simulink model "model"  (R2017a)
settings: Solver=ode45  StartTime=0.0  StopTime=25  MaxStep=0.005  MinStep=0.00001  RelTol=1e-4
settings Model: Creator=wangc  LastModifiedBy=wangc

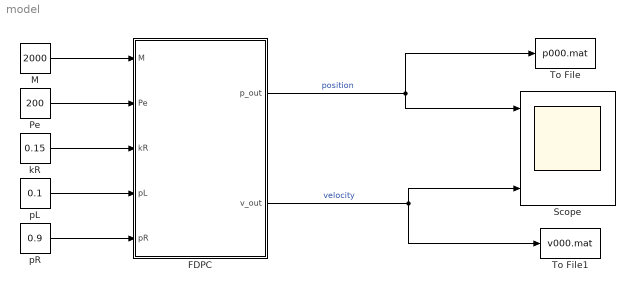
== system model ==
  FDPC : Stateflow chart  TreatAsAtomicUnit=on
  M : Constant  Value=2000
  Pe : Constant  Value=200
  Scope : Scope  NumInputPorts=3
  To File : ToFile  Filename=p000.mat  MatrixName=p  SaveFormat=Timeseries
  To File1 : ToFile  Filename=v000.mat  MatrixName=v  SaveFormat=Timeseries
  kR : Constant  Value=0.15
  pL : Constant  Value=0.1
  pR : Constant  Value=0.9
  wires:
  FDPC/2(v_out) -> To File1/1, Scope/3  "velocity"
  FDPC/1(p_out) -> To File/1, Scope/1  "position"
  M/1 -> FDPC/1(M)
  Pe/1 -> FDPC/2(Pe)
  kR/1 -> FDPC/3(kR)
  pL/1 -> FDPC/4(pL)
  pR/1 -> FDPC/5(pR)

== stateflow chart model/FDPC ==
  settings: updateMethod=CONTINUOUS  executeAtInitialization=1  initializeOutput=1
  state drivf=driv(vt, dirt, Pet) [function]
    (default) -> (junction 54) : {drivf=0.95*Pet*dirt/(vt+0.00005);}
  state system_mode_1 [group]
    state drivL
      du:
      % derivatives
      p_dot = v;
      v_dot = driv(v, dir, Pe)/M-9.81*kR;
      % outputs
      p_out = p;
      v_out = v;
    state drivL1
      du:
      % derivatives
      p_dot = v;
      v_dot = driv(-1*v, dir, Pe)/M+9.81*kR;
      % outputs
      p_out = p;
      v_out = v;
    drivL1 -> drivL [order 1] : [v>=0]
  state system_mode_3 [group]
    state drivR
      du:
      % derivatives
      p_dot = v;
      v_dot = driv(v, dir, Pe)/M-9.81*kR;
      % outputs
      p_out = p;
      v_out = v;
    state drivR1
      du:
      % derivatives
      p_dot = v;
      v_dot = driv(-1*v, dir, Pe)/M+9.81*kR;
      % outputs
      p_out = p;
      v_out = v;
    drivR -> drivR1 [order 2] : [v<=0]
  state system_mode_2 [group]
    state drivLR
      du:
      % derivatives
      p_dot = v;
      v_dot = 2*driv(v, dir, Pe)/M-9.81*kR;
      % outputs
      p_out = p;
      v_out = v;
    state drivLR1
      du:
      % derivatives
      p_dot = v;
      v_dot = 2*driv(-1*v, dir, Pe)/M+9.81*kR;
      % outputs
      p_out = p;
      v_out = v;
  (default) -> drivL : {
      | p = 0.25;
      | v = 0.000001;
      | dir=1;
      | }
  drivR -> drivR [order 1] : [p>=pR-0.25]
      | {dir=-1;}
  drivLR -> drivR : [p>0.55]
  drivL -> drivLR : [ p >=0.45 ]
  drivL1 -> drivL1 [order 2] : [p<=pL+0.25]
      | {dir=1;}
  drivR1 -> drivLR1 : [p<=0.55]
  drivLR1 -> drivL1 : [p<0.45]
  data: vt function_input double; dirt function_input double; Pet function_input double; drivf function_output double; p_out output double size=1; p local double; v local double; v_out output double size=1; M input; Pe input; kR input; pL input; pR input; dir local double
  data p settings: updateMethod=SF_CONTINUOUS_TIME_DATA
  data v settings: updateMethod=SF_CONTINUOUS_TIME_DATA
